simulink model "PowerConverters"  (R2024b)
settings: Solver=FixedStepAuto  StartTime=0.0  StopTime=tfinal  RelTol=1e-4  EnableMultiTasking=on
PreLoadFcn:
  | PowerConvertersInit;
InitFcn:
  | PowerConvertersInit;
values from neighbouring files (symbols this model uses):
  AmplitudeVar_Buck = 50    [PowerConvertersInit.m]
  Cfilter = 200e-6    (= 0.0002)    [PowerConvertersInit.m]
  Clink_3L = Pnom_dc_3L*H_3L*2 /Vnom_dc_3L^2    (= 0.0666666666667)    [PowerConvertersInit.m]
  Clink_stat = Pnom_stat*H_stat*2 /Vnom_dc_stat^2    (= 0.0115740740741)    [PowerConvertersInit.m]
  D_Boost = 0.8    [PowerConvertersInit.m]
  D_Buck = 0.55    [PowerConvertersInit.m]
  Fnom = 60    [PowerConvertersInit.m]
  FrequencyVar_Buck = 5    [PowerConvertersInit.m]
  Fsys_FB = 50    [PowerConvertersInit.m]
  J = 10    [PowerConvertersInit.m]
  Ki_Ireg_3L = 8    [PowerConvertersInit.m]
  Ki_Ireg_motor = 0.25    [PowerConvertersInit.m]
  Ki_Ireg_stat = 80    [PowerConvertersInit.m]
  Ki_VDCreg_3L = 275    [PowerConvertersInit.m]
  Ki_VDCreg_stat = 800    [PowerConvertersInit.m]
  Ki_wreg_motor = 50    [PowerConvertersInit.m]
  Kp_Ireg_3L = 0.2/2    (= 0.1)    [PowerConvertersInit.m]
  Kp_Ireg_motor = 0.0015    [PowerConvertersInit.m]
  Kp_Ireg_stat = 0.35    [PowerConvertersInit.m]
  Kp_VDCreg_3L = 2.5    [PowerConvertersInit.m]
  Kp_VDCreg_stat = 10    [PowerConvertersInit.m]
  Kp_wreg_motor = 15    [PowerConvertersInit.m]
  Lchoke_Boost = 1e-3    (= 0.001)    [PowerConvertersInit.m]
  Lchoke_Buck = 5e-3    (= 0.005)    [PowerConvertersInit.m]
  Lchoke_FB = 1e-3    (= 0.001)    [PowerConvertersInit.m]
  Lff_3L = Lxfo_3L    (= 0.1)    [PowerConvertersInit.m]
  Lff_stat = Lxfo_Tr_stat+0.06*2    (= 0.18)    [PowerConvertersInit.m]
  Limit_Ireg_motor = [1, 0]    [PowerConvertersInit.m]
  Limit_wreg_motor = [1000, -1000]    [PowerConvertersInit.m]
  LimitL_Ireg_3L = -1.5    [PowerConvertersInit.m]
  LimitL_Ireg_stat = -1.5    [PowerConvertersInit.m]
  LimitL_VDCreg_3L = -1.5    [PowerConvertersInit.m]
  LimitL_VDCreg_stat = -1.5    [PowerConvertersInit.m]
  LimitU_Ireg_3L = 1.5    [PowerConvertersInit.m]
  LimitU_Ireg_stat = 1.5    [PowerConvertersInit.m]
  LimitU_VDCreg_3L = 1.5    [PowerConvertersInit.m]
  LimitU_VDCreg_stat = 1.5    [PowerConvertersInit.m]
  Lm_Tr_stat = 200    [PowerConvertersInit.m]
  Lstat = 0.1*Lbase_sec    (= 0.000671434916169)    [PowerConvertersInit.m]
  Lxfo_3L = 0.10    (= 0.1)    [PowerConvertersInit.m]
  Lxfo_Tr_stat = 0.06    [PowerConvertersInit.m]
  m_FB = 0.9    [PowerConvertersInit.m]
  m_HB = 1    [PowerConvertersInit.m]
  Pnom_3L = Pnom_dc_3L    (= 1000000)    [PowerConvertersInit.m]
  Pnom_dc_3L = 1e6    (= 1000000)    [PowerConvertersInit.m]
  Pnom_stat = 2e6    (= 2000000)    [PowerConvertersInit.m]
  Psc_grid = 100e6    (= 100000000)    [PowerConvertersInit.m]
  R_DCsrc = 0.5    [PowerConvertersInit.m]
  RateLimit_Iref_motor = 20000    [PowerConvertersInit.m]
  RateLimit_Qstat = Fnom*2    (= 120)    [PowerConvertersInit.m]
  RateLimit_wref_motor = 2000    [PowerConvertersInit.m]
  Rchoke_Boost = 50e-3    (= 0.05)    [PowerConvertersInit.m]
  Rchoke_Buck = 10e-3    (= 0.01)    [PowerConvertersInit.m]
  Rchoke_FB = 50e-3    (= 0.05)    [PowerConvertersInit.m]
  Rff_3L = Rxfo_3L    (= 0.00333333333333)    [PowerConvertersInit.m]
  Rff_stat = Rxfo_Tr_stat+0.06/100*2    (= 0.0032)    [PowerConvertersInit.m]
  Rfilter = 1/(Cfilter*377)/50    (= 0.26525198939)    [PowerConvertersInit.m]
  Rload_Buck = 0.1    [PowerConvertersInit.m]
  Rm_Tr_stat = 200    [PowerConvertersInit.m]
  Rstat = Lstat*(2*pi*Fnom)/100    (= 0.00253125)    [PowerConvertersInit.m]
  Rxfo_3L = 0.10/30    (= 0.00333333333333)    [PowerConvertersInit.m]
  Rxfo_Tr_stat = 0.06/30    (= 0.002)    [PowerConvertersInit.m]
  Tload = 1000    [PowerConvertersInit.m]
  Ts_Control = 50e-6    (= 5e-05)    [PowerConvertersInit.m]
  Ts_Power = 1e-7    (= 1e-07)    [PowerConvertersInit.m]
  Ts_PWM = 1e-7    (= 1e-07)    [PowerConvertersInit.m]
  V_DCsrc = 500    [PowerConvertersInit.m]
  Vload_Buck = 500    [PowerConvertersInit.m]
  Vnom_dc_3L = 1000    [PowerConvertersInit.m]
  Vnom_dc_stat = 2400    [PowerConvertersInit.m]
  Vnom_grid = 25e3    (= 25000)    [PowerConvertersInit.m]
  Vnom_prim_3L = Vnom_grid    (= 25000)    [PowerConvertersInit.m]
  Vnom_prim_stat = Vnom_grid    (= 25000)    [PowerConvertersInit.m]
  Vnom_sec_3L = 0.5*Vnom_dc_3L/sqrt(2)*sqrt(3)*m_nom_3L    [PowerConvertersInit.m]
  Vnom_sec_stat = 1800*1.25    (= 2250)    [PowerConvertersInit.m]
  wref_Initial = w_Initial*30/pi    (= 1200)    [PowerConvertersInit.m]
undefined symbols (not defined in the file or in its folder): D1, Delta, DiscIntNeverNeededParam
libraries: spsSeriesRLCBranchLib x21, spsVoltageMeasurementLib x9, spsPWMGeneratorPulseAveragingLib x7, spsCurrentMeasurementLib x5, spsMeanLib x5, spsPWMGenerator2LevelLib x4, spsPWMGeneratorDCDCLib x4, spsabctodq0Lib x4, spsSecondOrderFilterLib x4, spsLinearTransformerLib x3, spsThreePhaseVIMeasurementLib x3, spsSeriesRLCLoadLib x2
(part 2 of 2)

== system PowerConverters/Control Systems/PWM Gen Boost ==
  Select : Inport
  D : Inport  Port=2
  PWM Gen : Subsystem
  Switch1 : Switch  Threshold=1.5  SaturateOnIntegerOverflow=off  InputSameDT=off
  g : Outport  VectorParamsAs1DForOutWhenUnconnected=off
  wires:
  D/1 -> PWM Gen/1(D)
  Select/1 -> Switch1/2, PWM Gen/Enable
  Switch1/1 -> g/1
  PWM Gen/1(g) -> Switch1/3
  PWM Gen/2(g_Pavg) -> Switch1/1

== system PowerConverters/Control Systems/PWM Gen Buck ==
  Select : Inport
  D : Inport  Port=2
  PWM Gen : Subsystem
  Switch1 : Switch  Threshold=1.5  SaturateOnIntegerOverflow=off  InputSameDT=off
  g : Outport  VectorParamsAs1DForOutWhenUnconnected=off
  wires:
  PWM Gen/2(g_Pavg) -> Switch1/1
  PWM Gen/1(g) -> Switch1/3
  Switch1/1 -> g/1
  Select/1 -> PWM Gen/Enable, Switch1/2
  D/1 -> PWM Gen/1(D)

== system PowerConverters/Control Systems/PWM Gen FB ==
  Select : Inport
  Uref : Inport  Port=2
  PWM gen : Subsystem
  Switch1 : Switch  Threshold=1.5  SaturateOnIntegerOverflow=off  InputSameDT=off
  g : Outport  VectorParamsAs1DForOutWhenUnconnected=off
  wires:
  PWM gen/1(g) -> Switch1/3
  Switch1/1 -> g/1
  Select/1 -> PWM gen/Enable, Switch1/2
  Uref/1 -> PWM gen/1(Uref)
  PWM gen/2(g_Pavg) -> Switch1/1

== system PowerConverters/Control Systems/PWM Gen HB ==
  Select : Inport
  Uref : Inport  Port=2
  Subsystem : Subsystem
  Switch1 : Switch  Threshold=1.5  SaturateOnIntegerOverflow=off  InputSameDT=off
  g : Outport  VectorParamsAs1DForOutWhenUnconnected=off
  wires:
  Uref/1 -> Subsystem/1(Uref)
  Select/1 -> Switch1/2, Subsystem/Enable
  Switch1/1 -> g/1
  Subsystem/1(g) -> Switch1/3
  Subsystem/2(g_Pavg) -> Switch1/1

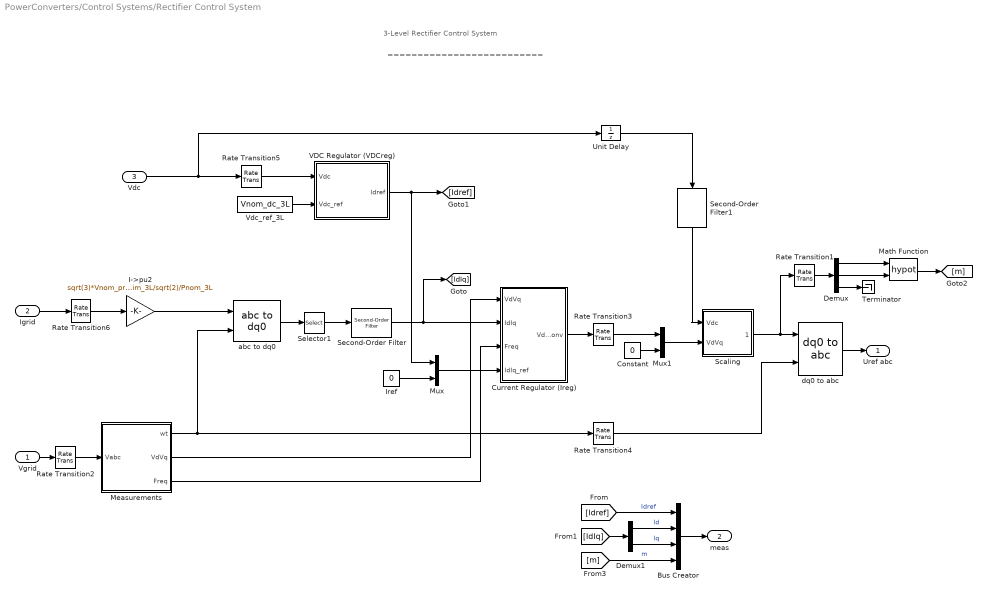
== system PowerConverters/Control Systems/Rectifier Control System ==
  note: 3-Level Rectifier Control System
  note: ==========================
  Vgrid : Inport  PortDimensions=3
  Igrid : Inport  Port=2  PortDimensions=3
  Vdc : Inport  Port=3
  Bus Creator : BusCreator  Inputs=4
  Constant : Constant  Value=0
  Current Regulator (Ireg) : Subsystem
  Demux : Demux  Outputs=3
  Demux1 : Demux  Outputs=2
  I->pu2 : Gain  Gain=sqrt(3)*Vnom_prim_3L/sqrt(2)/Pnom_3L  SaturateOnIntegerOverflow=on  OutDataTypeStr=Inherit: Same as input  ParamDataTypeStr=Inherit: Same as input
  Iref : Constant  Value=0
  Math Function : Math  Operator=hypot  SignedPower=on
  Measurements : Subsystem
  Mux : Mux  Inputs=2
  Mux1 : Mux  Inputs=[2 1]
  Rate Transition{1..2,5..6} (4 alike) : RateTransition  OutPortSampleTime=Ts_Control
  Rate Transition3 : RateTransition  OutPortSampleTime=Ts_PWM
  Rate Transition4 : RateTransition  OutPortSampleTime=Ts_PWM
  Scaling : Subsystem
  Second-Order Filter : spsSecondOrderFilterLib/Second-Order Filter  FilterType=Lowpass  Fo=Freq_Filter  Zeta=1  Ts=Ts_Control  Initialize=off  Vac_Init="[0,  0,  60]"  Vdc_Init=0  PlotResponse=off  FreqRange=[0, 500, 1]
  Second-Order Filter1 : spsSecondOrderFilterLib/Second-Order Filter  FilterType=Lowpass  Fo=Freq_Filter  Zeta=1  Ts=Ts_PWM  Initialize=off  Vac_Init="[0,  0,  60]"  Vdc_Init=0  PlotResponse=off  FreqRange=[0, 500, 1]
  Selector1 : Selector  InputPortWidth=3  IndexOptions=Index vector (dialog)  Indices=[1 2]  OutputSizes=1
  Terminator : Terminator
  Unit Delay : UnitDelay  SampleTime=Ts_PWM  HasFrameUpgradeWarning=on
  VDC Regulator (VDCreg) : Subsystem
  Vdc_ref_3L : Constant  Value=Vnom_dc_3L
  abc to dq0 : spsabctodq0Lib/abc to dq0  Alignment=90 degrees behind phase A axis
  dq0 to abc : spsdq0toabcLib/dq0 to abc  Alignment=90 degrees behind phase A axis
  Uref abc : Outport  VectorParamsAs1DForOutWhenUnconnected=off
  meas : Outport  Port=2  VectorParamsAs1DForOutWhenUnconnected=off
  wires:
  Selector1/1 -> Second-Order Filter/1
  I->pu2/1 -> abc to dq0/1
  Igrid/1 -> Rate Transition6/1
  abc to dq0/1 -> Selector1/1
  VDC Regulator (VDCreg)/1(Idref) -> [Idref], Mux/1
  Scaling/1(VdVq*) -> dq0 to abc/1, Rate Transition1/1
  Mux1/1 -> Scaling/2(VdVq)
  Mux/1 -> Current Regulator (Ireg)/4(IdIq_ref)
  Demux/3 -> Terminator/1
  Demux/2 -> Math Function/2
  Demux/1 -> Math Function/1
  Constant/1 -> Mux1/2
  Rate Transition3/1 -> Mux1/1
  Rate Transition4/1 -> dq0 to abc/2
  Current Regulator (Ireg)/1(VdVq_conv) -> Rate Transition3/1
  dq0 to abc/1 -> Uref abc/1
  Vgrid/1 -> Rate Transition2/1
  Rate Transition2/1 -> Measurements/1(Vabc)
  Rate Transition6/1 -> I->pu2/1
  Measurements/1(wt) -> Rate Transition4/1, abc to dq0/2
  Measurements/2(VdVq) -> Current Regulator (Ireg)/1(VdVq)
  Measurements/3(Freq) -> Current Regulator (Ireg)/3(Freq)
  Iref/1 -> Mux/2
  Vdc_ref_3L/1 -> VDC Regulator (VDCreg)/2(Vdc_ref)
  [Idref] -> Bus Creator/1  "Idref"
  Demux1/1 -> Bus Creator/2  "Id"
  Demux1/2 -> Bus Creator/3  "Iq"
  [m] -> Bus Creator/4  "m"
  [IdIq] -> Demux1/1
  Bus Creator/1 -> meas/1
  Math Function/1 -> [m]
  Rate Transition5/1 -> VDC Regulator (VDCreg)/1(Vdc)
  Rate Transition1/1 -> Demux/1
  Vdc/1 -> Unit Delay/1, Rate Transition5/1
  Unit Delay/1 -> Second-Order Filter1/1
  Second-Order Filter/1 -> [IdIq], Current Regulator (Ireg)/2(IdIq)
  Second-Order Filter1/1 -> Scaling/1(Vdc)

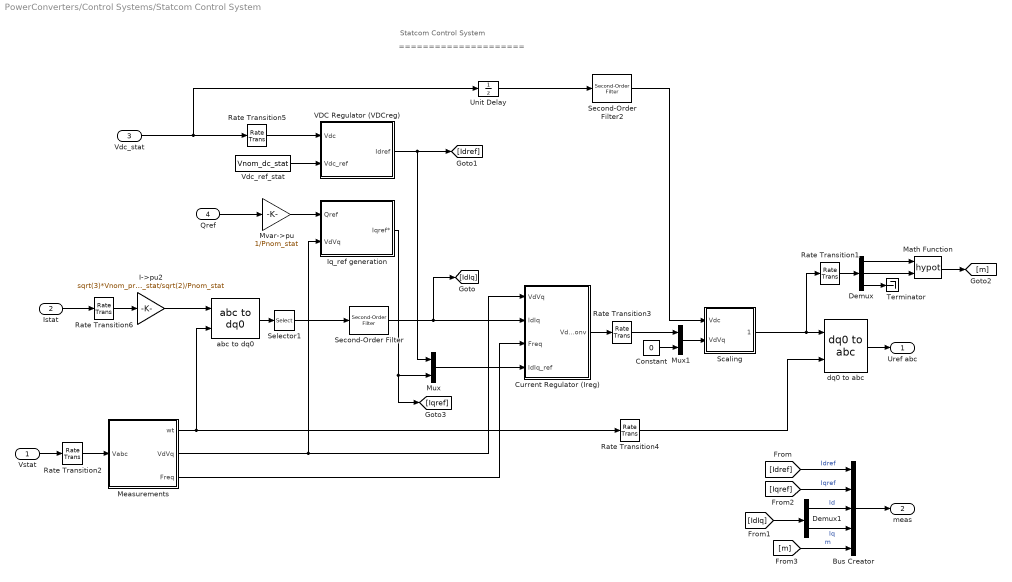
== system PowerConverters/Control Systems/Statcom Control System ==
  note: Statcom Control System
  note: =====================
  Vstat : Inport  PortDimensions=3
  Istat : Inport  Port=2  PortDimensions=3
  Vdc_stat : Inport  Port=3
  Qref : Inport  Port=4  PortDimensions=1
  Bus Creator : BusCreator  Inputs=5
  Constant : Constant  Value=0
  Current Regulator (Ireg) : Subsystem
  Demux : Demux  Outputs=3
  Demux1 : Demux  Outputs=2
  I->pu2 : Gain  Gain=sqrt(3)*Vnom_prim_stat/sqrt(2)/Pnom_stat  SaturateOnIntegerOverflow=on  OutDataTypeStr=Inherit: Same as input  ParamDataTypeStr=Inherit: Same as input
  Iq_ref generation : Subsystem
  Math Function : Math  Operator=hypot  SignedPower=on
  Measurements : Subsystem
  Mux : Mux  Inputs=2
  Mux1 : Mux  Inputs=[2 1]
  Mvar->pu : Gain  Gain=1/Pnom_stat  SaturateOnIntegerOverflow=on  OutDataTypeStr=Inherit: Same as input  ParamDataTypeStr=Inherit: Same as input
  Rate Transition{1..2,5..6} (4 alike) : RateTransition  OutPortSampleTime=Ts_Control
  Rate Transition3 : RateTransition  OutPortSampleTime=Ts_PWM
  Rate Transition4 : RateTransition  OutPortSampleTime=Ts_PWM
  Scaling : Subsystem
  Second-Order Filter : spsSecondOrderFilterLib/Second-Order Filter  FilterType=Lowpass  Fo=Freq_Filter_stat  Zeta=1  Ts=Ts_Control  Initialize=off  Vac_Init="[0,  0,  60]"  Vdc_Init=0  PlotResponse=off  FreqRange=[0, 500, 1]
  Second-Order Filter2 : spsSecondOrderFilterLib/Second-Order Filter  FilterType=Lowpass  Fo=Freq_Filter_stat  Zeta=1  Ts=Ts_PWM  Initialize=off  Vac_Init="[0,  0,  60]"  Vdc_Init=0  PlotResponse=off  FreqRange=[0, 500, 1]
  Selector1 : Selector  InputPortWidth=3  IndexOptions=Index vector (dialog)  Indices=[1 2]  OutputSizes=1
  Terminator : Terminator
  Unit Delay : UnitDelay  SampleTime=Ts_PWM  HasFrameUpgradeWarning=on
  VDC Regulator (VDCreg) : Subsystem
  Vdc_ref_stat : Constant  Value=Vnom_dc_stat
  abc to dq0 : spsabctodq0Lib/abc to dq0  Alignment=90 degrees behind phase A axis
  dq0 to abc : spsdq0toabcLib/dq0 to abc  Alignment=90 degrees behind phase A axis
  Uref abc : Outport  VectorParamsAs1DForOutWhenUnconnected=off
  meas : Outport  Port=2  VectorParamsAs1DForOutWhenUnconnected=off
  wires:
  Mvar->pu/1 -> Iq_ref generation/1(Qref)
  Second-Order Filter2/1 -> Scaling/1(Vdc)
  Qref/1 -> Mvar->pu/1
  Iq_ref generation/1(Iqref*) -> [Iqref], Mux/2
  Vdc_ref_stat/1 -> VDC Regulator (VDCreg)/2(Vdc_ref)
  VDC Regulator (VDCreg)/1(Idref) -> [Idref], Mux/1
  [m] -> Bus Creator/5  "m"
  Demux1/2 -> Bus Creator/4  "Iq"
  Demux1/1 -> Bus Creator/3  "Id"
  [Iqref] -> Bus Creator/2  "Iqref"
  [Idref] -> Bus Creator/1  "Idref"
  Selector1/1 -> Second-Order Filter/1
  I->pu2/1 -> abc to dq0/1
  Istat/1 -> Rate Transition6/1
  abc to dq0/1 -> Selector1/1
  Scaling/1(VdVq*) -> dq0 to abc/1, Rate Transition1/1
  Mux1/1 -> Scaling/2(VdVq)
  Mux/1 -> Current Regulator (Ireg)/4(IdIq_ref)
  Demux/3 -> Terminator/1
  Demux/2 -> Math Function/2
  Demux/1 -> Math Function/1
  Constant/1 -> Mux1/2
  Rate Transition3/1 -> Mux1/1
  Rate Transition4/1 -> dq0 to abc/2
  Current Regulator (Ireg)/1(VdVq_conv) -> Rate Transition3/1
  dq0 to abc/1 -> Uref abc/1
  Vstat/1 -> Rate Transition2/1
  Rate Transition2/1 -> Measurements/1(Vabc)
  Rate Transition6/1 -> I->pu2/1
  Measurements/1(wt) -> Rate Transition4/1, abc to dq0/2
  Measurements/2(VdVq) -> Iq_ref generation/2(VdVq), Current Regulator (Ireg)/1(VdVq)
  Measurements/3(Freq) -> Current Regulator (Ireg)/3(Freq)
  [IdIq] -> Demux1/1
  Bus Creator/1 -> meas/1
  Math Function/1 -> [m]
  Rate Transition5/1 -> VDC Regulator (VDCreg)/1(Vdc)
  Rate Transition1/1 -> Demux/1
  Vdc_stat/1 -> Unit Delay/1, Rate Transition5/1
  Second-Order Filter/1 -> [IdIq], Current Regulator (Ireg)/2(IdIq)
  Unit Delay/1 -> Second-Order Filter2/1

== system PowerConverters/Control Systems/DC Motor Control/Current regulator Ireg_motor ==
  Error : Inport  SampleTime=Ts
  Discrete-Time Integrator : DiscreteIntegrator  InitialCondition=Init  SampleTime=Ts  LimitOutput=on  UpperSaturationLimit=UpperLimit  LowerSaturationLimit=LowerLimit  ICPrevOutput=DiscIntNeverNeededParam  ICPrevScaledInput=DiscIntNeverNeededParam
  Kp4 : Gain  Gain=Kp  SaturateOnIntegerOverflow=on  SampleTime=Ts  OutDataTypeStr=Inherit: Same as input  ParamDataTypeStr=Inherit: Same as input
  Kp5 : Gain  Gain=Ki  SaturateOnIntegerOverflow=on  SampleTime=Ts  OutDataTypeStr=Inherit: Same as input  ParamDataTypeStr=Inherit: Same as input
  Saturation2 : Saturate  UpperLimit=UpperLimit  LowerLimit=LowerLimit  SampleTime=Ts
  Sum6 : Sum  InputSameDT=on  SaturateOnIntegerOverflow=on  SampleTime=Ts  OutDataTypeStr=Inherit: Same as first input
  Zero-Order Hold : ZeroOrderHold  SampleTime=Ts
  Out : Outport  SampleTime=Ts  InitialOutput=0  VectorParamsAs1DForOutWhenUnconnected=off
  wires:
  Zero-Order Hold/1 -> Sum6/1
  Saturation2/1 -> Out/1
  Discrete-Time Integrator/1 -> Sum6/2
  Kp4/1 -> Zero-Order Hold/1
  Kp5/1 -> Discrete-Time Integrator/1
  Sum6/1 -> Saturation2/1
  Error/1 -> Kp5/1, Kp4/1

== system PowerConverters/Control Systems/DC Motor Control/Speed Regulator wreg ==
  Error : Inport  SampleTime=Ts
  Discrete-Time Integrator : DiscreteIntegrator  InitialCondition=Init  SampleTime=Ts  LimitOutput=on  UpperSaturationLimit=UpperLimit  LowerSaturationLimit=LowerLimit  ICPrevOutput=DiscIntNeverNeededParam  ICPrevScaledInput=DiscIntNeverNeededParam
  Kp4 : Gain  Gain=Kp  SaturateOnIntegerOverflow=on  SampleTime=Ts  OutDataTypeStr=Inherit: Same as input  ParamDataTypeStr=Inherit: Same as input
  Kp5 : Gain  Gain=Ki  SaturateOnIntegerOverflow=on  SampleTime=Ts  OutDataTypeStr=Inherit: Same as input  ParamDataTypeStr=Inherit: Same as input
  Saturation2 : Saturate  UpperLimit=UpperLimit  LowerLimit=LowerLimit  SampleTime=Ts
  Sum6 : Sum  InputSameDT=on  SaturateOnIntegerOverflow=on  SampleTime=Ts  OutDataTypeStr=Inherit: Same as first input
  Zero-Order Hold : ZeroOrderHold  SampleTime=Ts
  Out : Outport  SampleTime=Ts  InitialOutput=0  VectorParamsAs1DForOutWhenUnconnected=off
  wires:
  Zero-Order Hold/1 -> Sum6/1
  Saturation2/1 -> Out/1
  Discrete-Time Integrator/1 -> Sum6/2
  Kp4/1 -> Zero-Order Hold/1
  Kp5/1 -> Discrete-Time Integrator/1
  Sum6/1 -> Saturation2/1
  Error/1 -> Kp5/1, Kp4/1

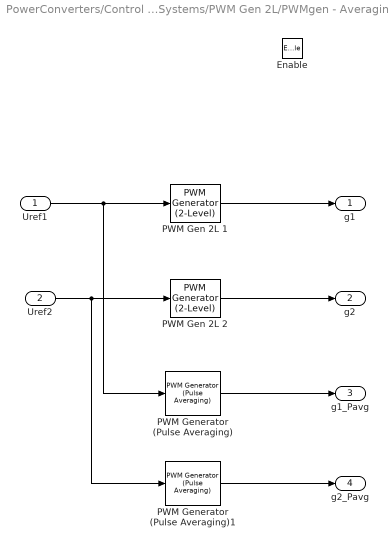
== system PowerConverters/Control Systems/PWM Gen 2L/PWMgen - Averaging ==
  Uref1 : Inport
  Uref2 : Inport  Port=2
  Enable : EnablePort
  PWM Gen 2L 1 : spsPWMGenerator2LevelLib/PWM Generator (2-Level)  ModulatorType=Three-phase bridge (6 pulses)  ModulatorMode=Unsynchronized  Fc=Fc_stat  Pc=90  nF=27  MinMax="[ -1  1 ]"  SamplingTechnique=Natural  ModulatingSignals=off  m=0.8  Freq=60  Phase=0  Ts=Ts_PWM  ShowCarrierOutport=off
  PWM Gen 2L 2 : spsPWMGenerator2LevelLib/PWM Generator (2-Level)  ModulatorType=Three-phase bridge (6 pulses)  ModulatorMode=Unsynchronized  Fc=Fc_stat  Pc=90  nF=27  MinMax="[ -1  1 ]"  SamplingTechnique=Natural  ModulatingSignals=off  m=0.8  Freq=60  Phase=0  Ts=Ts_PWM  ShowCarrierOutport=off
  PWM Generator (Pulse Averaging) : spsPWMGeneratorPulseAveragingLib/PWM Generator (Pulse Averaging)  GeneratorType=Two-level, three-phase  Fc=Fc_stat  InitialPhase=90  Ts=Ts_PWM
  PWM Generator (Pulse Averaging)1 : spsPWMGeneratorPulseAveragingLib/PWM Generator (Pulse Averaging)  GeneratorType=Two-level, three-phase  Fc=Fc_stat  InitialPhase=90  Ts=Ts_PWM
  g1 : Outport  VectorParamsAs1DForOutWhenUnconnected=off
  g2 : Outport  Port=2  VectorParamsAs1DForOutWhenUnconnected=off
  g1_Pavg : Outport  Port=3  VectorParamsAs1DForOutWhenUnconnected=off
  g2_Pavg : Outport  Port=4  VectorParamsAs1DForOutWhenUnconnected=off
  wires:
  Uref1/1 -> PWM Generator (Pulse Averaging)/1, PWM Gen 2L 1/1
  Uref2/1 -> PWM Generator (Pulse Averaging)1/1, PWM Gen 2L 2/1
  PWM Gen 2L 1/1 -> g1/1
  PWM Gen 2L 2/1 -> g2/1
  PWM Generator (Pulse Averaging)/1 -> g1_Pavg/1
  PWM Generator (Pulse Averaging)1/1 -> g2_Pavg/1

== system PowerConverters/Control Systems/PWM Gen 2Q/Subsystem ==
  D : Inport
  Enable : EnablePort
  Logical Operator : Logic  Operator=NOT  AllPortsSameDT=off  OutDataTypeStr=float('double')
  Mux : Mux  Inputs=2
  "PWM Gen 2Q " : spsPWMGeneratorDCDCLib/PWM Generator (DC-DC)  Fsw=Fc_motor  Ts=Ts_PWM
  PWM Generator (Pulse Averaging) : spsPWMGeneratorPulseAveragingLib/PWM Generator (Pulse Averaging)  GeneratorType=Two-quadrant  Fc=Fc_motor  InitialPhase=0  Ts=Ts_PWM
  g : Outport  VectorParamsAs1DForOutWhenUnconnected=off
  g_Pavg : Outport  Port=2  VectorParamsAs1DForOutWhenUnconnected=off
  wires:
  Mux/1 -> g/1
  Logical Operator/1 -> Mux/2
  D/1 -> PWM Generator (Pulse Averaging)/1, "PWM Gen 2Q "/1
  "PWM Gen 2Q "/1 -> Logical Operator/1, Mux/1
  PWM Generator (Pulse Averaging)/1 -> g_Pavg/1

== system PowerConverters/Control Systems/PWM Gen 3L/PWMgen - Averaging ==
  Uref : Inport
  Enable : EnablePort
  PWM Generator (Pulse Averaging) : spsPWMGeneratorPulseAveragingLib/PWM Generator (Pulse Averaging)  GeneratorType=Three-level, three-phase  Fc=Fc_3L  InitialPhase=0  Ts=Ts_PWM
  Subsystem : Subsystem
  Pavg : Outport  VectorParamsAs1DForOutWhenUnconnected=off
  P : Outport  Port=2  VectorParamsAs1DForOutWhenUnconnected=off
  wires:
  Uref/1 -> Subsystem/1(Uref), PWM Generator (Pulse Averaging)/1
  PWM Generator (Pulse Averaging)/1 -> Pavg/1
  Subsystem/1(P) -> P/1

== system PowerConverters/Control Systems/PWM Gen Boost/PWM Gen ==
  D : Inport
  Enable : EnablePort
  "PWM Gen Buck " : spsPWMGeneratorDCDCLib/PWM Generator (DC-DC)  Fsw=Fc_Boost  Ts=Ts_PWM
  PWM Generator (DC-DC) : spsPWMGeneratorDCDCLib/PWM Generator (DC-DC)  Fsw=Fc_Boost  Ts=Ts_PWM
  g : Outport  VectorParamsAs1DForOutWhenUnconnected=off
  g_Pavg : Outport  Port=2  VectorParamsAs1DForOutWhenUnconnected=off
  wires:
  "PWM Gen Buck "/1 -> g/1
  D/1 -> PWM Generator (DC-DC)/1, "PWM Gen Buck "/1
  PWM Generator (DC-DC)/1 -> g_Pavg/1

== system PowerConverters/Control Systems/PWM Gen Buck/PWM Gen ==
  D : Inport
  Enable : EnablePort
  "PWM Gen Buck " : spsPWMGeneratorDCDCLib/PWM Generator (DC-DC)  Fsw=Fc_Buck  Ts=Ts_PWM
  PWM Generator (Pulse Averaging) : spsPWMGeneratorPulseAveragingLib/PWM Generator (Pulse Averaging)  GeneratorType=Two-quadrant  Fc=Fc_Buck  InitialPhase=0  Ts=Ts_PWM
  Selector : Selector  InputPortWidth=2  IndexOptions=Index vector (dialog)  Indices=1  OutputSizes=1
  g : Outport  VectorParamsAs1DForOutWhenUnconnected=off
  g_Pavg : Outport  Port=2  VectorParamsAs1DForOutWhenUnconnected=off
  wires:
  PWM Generator (Pulse Averaging)/1 -> Selector/1
  D/1 -> PWM Generator (Pulse Averaging)/1, "PWM Gen Buck "/1
  "PWM Gen Buck "/1 -> g/1
  Selector/1 -> g_Pavg/1

== system PowerConverters/Control Systems/PWM Gen FB/PWM gen ==
  Uref : Inport
  Enable : EnablePort
  PWM Gen FB : spsPWMGenerator2LevelLib/PWM Generator (2-Level)  ModulatorType=Single-phase full-bridge (4 pulses)  ModulatorMode=Unsynchronized  Fc=Fc_FB  Pc=90  nF=27  MinMax="[ -1  1 ]"  SamplingTechnique=Natural  ModulatingSignals=off  m=0.8  Freq=60  Phase=0  Ts=Ts_PWM  ShowCarrierOutport=off
  PWM Generator (Pulse Averaging) : spsPWMGeneratorPulseAveragingLib/PWM Generator (Pulse Averaging)  GeneratorType=Full-bridge, single phase  Fc=Fc_FB  InitialPhase=90  Ts=Ts_PWM
  g : Outport  VectorParamsAs1DForOutWhenUnconnected=off
  g_Pavg : Outport  Port=2  VectorParamsAs1DForOutWhenUnconnected=off
  wires:
  PWM Generator (Pulse Averaging)/1 -> g_Pavg/1
  PWM Gen FB/1 -> g/1
  Uref/1 -> PWM Generator (Pulse Averaging)/1, PWM Gen FB/1

== system PowerConverters/Control Systems/PWM Gen HB/Subsystem ==
  Uref : Inport
  Enable : EnablePort
  PWM Gen HB : spsPWMGenerator2LevelLib/PWM Generator (2-Level)  ModulatorType=Single-phase half-bridge (2 pulses)  ModulatorMode=Unsynchronized  Fc=Fc_HB  Pc=90  nF=27  MinMax="[ -1  1 ]"  SamplingTechnique=Natural  ModulatingSignals=off  m=0.8  Freq=60  Phase=0  Ts=Ts_PWM  ShowCarrierOutport=off
  PWM Generator (Pulse Averaging) : spsPWMGeneratorPulseAveragingLib/PWM Generator (Pulse Averaging)  GeneratorType=Full-bridge, single phase  Fc=Fc_HB  InitialPhase=0  Ts=Ts_PWM
  Selector : Selector  InputPortWidth=4  IndexOptions=Index vector (dialog)  Indices=[1,2]  OutputSizes=1
  g : Outport  VectorParamsAs1DForOutWhenUnconnected=off
  g_Pavg : Outport  Port=2  VectorParamsAs1DForOutWhenUnconnected=off
  wires:
  PWM Gen HB/1 -> g/1
  Selector/1 -> g_Pavg/1
  PWM Generator (Pulse Averaging)/1 -> Selector/1
  Uref/1 -> PWM Generator (Pulse Averaging)/1, PWM Gen HB/1

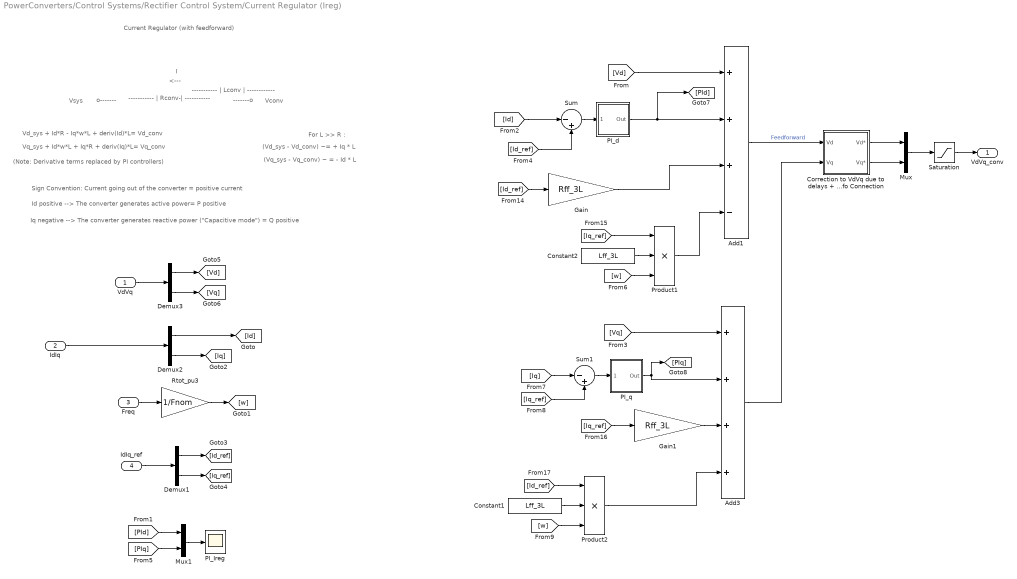
== system PowerConverters/Control Systems/Rectifier Control System/Current Regulator (Ireg) ==
  note: <---
  note: -------o
  note: Vconv
  note: -----------
      | | Lconv |
      | ------------
  note: ----
  note: -----------
      | | Rconv |
      | -----------
  note: For L >> R :
  note: (Vq_sys - Vq_conv) ~ = - Id * L
  note: (Vd_sys - Vd_conv) ~= + Iq * L
  note: Id positive --> The converter generates active power= P positive
  note: Iq negative --> The converter generates reactive power ("Capacitive mode") = Q positive
  note: Sign Convention: Current going out of the converter = positive current
  note: Current Regulator
      | (with feedforward)
  note: Vq_sys + Id*w*L + Iq*R + deriv(Iq)*L= Vq_conv
  note: Vd_sys + Id*R - Iq*w*L + deriv(Id)*L= Vd_conv
  note: (Note: Derivative terms replaced by PI controllers)
  note: Vsys
  note: o-------
  note: I
  VdVq : Inport  PortDimensions=2
  IdIq : Inport  Port=2  PortDimensions=2
  Freq : Inport  Port=3  PortDimensions=1
  IdIq_ref : Inport  Port=4  PortDimensions=2
  Add1 : Sum  Inputs=+++-
  Add3 : Sum  Inputs=++++
  Constant1 : Constant  Value=Lff_3L  SampleTime=Ts_Control
  Constant2 : Constant  Value=Lff_3L  SampleTime=Ts_Control
  Correction to VdVq due to delays + Transfo Connection : Subsystem
  Demux1 : Demux  Outputs=2
  Demux2 : Demux  Outputs=2
  Demux3 : Demux  Outputs=2
  Gain : Gain  Gain=Rff_3L
  Gain1 : Gain  Gain=Rff_3L
  Mux : Mux  Inputs=2
  Mux1 : Mux  Inputs=2
  PI_Ireg : Scope
  PI_d : Subsystem  DialogController=POWERSYS.PowerSysDialog  mask(Discrete PI Controller){Kp=Kp_Ireg_3L, Ki=Ki_Ireg_3L, Par_Limits=[ LimitU_Ireg_3L LimitL_Ireg_3L ], Init=0, Ts=Ts_Control}
      mask prompts: Kp "Proportional gain (Kp):"; Ki "Integral gain (Ki):"; Par_Limits "Output limits: [ Upper   Lower ]"; Init "Output initial value:"; Ts "Sample time:"
      mask help: This block implements a discrete PI controller.
      mask init:
      | UpperLimit=Par_Limits(1);
      | LowerLimit=Par_Limits(2);
      mask Display: disp('PI');
  PI_q : Subsystem  DialogController=POWERSYS.PowerSysDialog  mask(Discrete PI Controller){Kp=Kp_Ireg_3L, Ki=Ki_Ireg_3L, Par_Limits=[ LimitU_Ireg_3L LimitL_Ireg_3L ], Init=0, Ts=Ts_Control}
      mask prompts: Kp "Proportional gain (Kp):"; Ki "Integral gain (Ki):"; Par_Limits "Output limits: [ Upper   Lower ]"; Init "Output initial value:"; Ts "Sample time:"
      mask help: This block implements a discrete PI controller.
      mask init:
      | UpperLimit=Par_Limits(1);
      | LowerLimit=Par_Limits(2);
      mask Display: disp('PI');
  Product1 : Product  Inputs=3  RndMeth=Zero
  Product2 : Product  Inputs=3  RndMeth=Zero
  Rtot_pu3 : Gain  Gain=1/Fnom  SaturateOnIntegerOverflow=on  OutDataTypeStr=Inherit: Same as input  ParamDataTypeStr=Inherit: Same as input
  Saturation : Saturate  UpperLimit=LimitU_Ireg_3L  LowerLimit=LimitL_Ireg_3L
  Sum : Sum  Inputs=|-+
  Sum1 : Sum  Inputs=|-+
  VdVq_conv : Outport  VectorParamsAs1DForOutWhenUnconnected=off
  wires:
  Add3/1 -> Correction to VdVq due to delays + Transfo Connection/2(Vq)
  Add1/1 -> Correction to VdVq due to delays + Transfo Connection/1(Vd)  "Feedforward"
  PI_d/1(Out) -> [PId], Add1/2
  PI_q/1(Out) -> [PIq], Add3/2
  [Vd] -> Add1/1
  Product1/1 -> Add1/4
  Gain/1 -> Add1/3
  Gain1/1 -> Add3/3
  Product2/1 -> Add3/4
  [Vq] -> Add3/1
  Demux2/1 -> [Id]
  IdIq/1 -> Demux2/1
  [Id_ref] -> Product2/1
  [Iq_ref] -> Gain1/1
  [Iq_ref] -> Product1/1
  [Id_ref] -> Gain/1
  Saturation/1 -> VdVq_conv/1
  [Id] -> Sum/1
  [Iq] -> Sum1/1
  Demux2/2 -> [Iq]
  Correction to VdVq due to delays + Transfo Connection/2(Vq*) -> Mux/2
  Correction to VdVq due to delays + Transfo Connection/1(Vd*) -> Mux/1
  [PIq] -> Mux1/2
  [PId] -> Mux1/1
  [w] -> Product1/3
  Constant2/1 -> Product1/2
  [w] -> Product2/3
  Constant1/1 -> Product2/2
  Mux1/1 -> PI_Ireg/1
  [Iq_ref] -> Sum1/2
  Sum1/1 -> PI_q/1(Error)
  [Id_ref] -> Sum/2
  Sum/1 -> PI_d/1(Error)
  Mux/1 -> Saturation/1
  VdVq/1 -> Demux3/1
  Demux3/2 -> [Vq]
  Demux3/1 -> [Vd]
  IdIq_ref/1 -> Demux1/1
  Demux1/2 -> [Iq_ref]
  Demux1/1 -> [Id_ref]
  Rtot_pu3/1 -> [w]
  Freq/1 -> Rtot_pu3/1

== system PowerConverters/Control Systems/Rectifier Control System/Measurements ==
  Vabc : Inport  PortDimensions=3
  PLL (3ph) : spsPLL3phLib/PLL (3ph)  Fmin=45  Par_Init=[0, Fnom]  ParK=[180, 3200, 0]/2  TcD=1e-4  MaxRateChangeFreq=12  FilterCutOffFreq=25  Ts=Ts_Control  AGC=on
  Selector2 : Selector  InputPortWidth=3  IndexOptions=Index vector (dialog)  Indices=[1 2]  OutputSizes=1
  V->pu1 : Gain  Gain=1/(Vnom_prim_3L*sqrt(2)/sqrt(3))  SaturateOnIntegerOverflow=on  OutDataTypeStr=Inherit: Same as input  ParamDataTypeStr=Inherit: Same as input
  abc to dq1 : spsabctodq0Lib/abc to dq0  Alignment=90 degrees behind phase A axis
  wt : Outport  VectorParamsAs1DForOutWhenUnconnected=off
  VdVq : Outport  Port=2  VectorParamsAs1DForOutWhenUnconnected=off
  Freq : Outport  Port=3  VectorParamsAs1DForOutWhenUnconnected=off
  wires:
  Selector2/1 -> VdVq/1
  abc to dq1/1 -> Selector2/1
  PLL (3ph)/1 -> Freq/1
  V->pu1/1 -> PLL (3ph)/1, abc to dq1/1
  Vabc/1 -> V->pu1/1
  PLL (3ph)/2 -> wt/1, abc to dq1/2

== system PowerConverters/Control Systems/Rectifier Control System/Scaling ==
  Vdc : Inport
  VdVq : Inport  Port=2
  0.8 to 1.2 x Vnom_dc : Saturate  UpperLimit=1.5*Vnom_dc_3L  LowerLimit=0.5*Vnom_dc_3L
  Constant1 : Constant  Value=Vnom_sec_3L
  Gain1 : Gain  Gain=0.5/sqrt(2)*sqrt(3)
  Product : Product  Inputs=*/
  Product1 : Product  Inputs=**
  VdVq* : Outport  VectorParamsAs1DForOutWhenUnconnected=off
  wires:
  Product1/1 -> VdVq*/1
  VdVq/1 -> Product1/1
  Vdc/1 -> 0.8 to 1.2 x Vnom_dc/1
  Product/1 -> Product1/2
  0.8 to 1.2 x Vnom_dc/1 -> Gain1/1
  Gain1/1 -> Product/2
  Constant1/1 -> Product/1

== system PowerConverters/Control Systems/Rectifier Control System/VDC Regulator (VDCreg) ==
  Vdc : Inport  PortDimensions=1
  Vdc_ref : Inport  Port=2  PortDimensions=1
  Gain : Gain  Gain=1/(Vnom_dc_3L)
  PI_d : Subsystem  DialogController=POWERSYS.PowerSysDialog  mask(Discrete PI Controller){Kp=Kp_VDCreg_3L, Ki=Ki_VDCreg_3L, Par_Limits=[ LimitU_VDCreg_3L LimitL_VDCreg_3L ], Init=0, Ts=Ts_Control}
      mask prompts: Kp "Proportional gain (Kp):"; Ki "Integral gain (Ki):"; Par_Limits "Output limits: [ Upper   Lower ]"; Init "Output initial value:"; Ts "Sample time:"
      mask help: This block implements a discrete PI controller.
      mask init:
      | UpperLimit=Par_Limits(1);
      | LowerLimit=Par_Limits(2);
      mask Display: disp('PI');
  Sum : Sum  Inputs=|-+
  Idref : Outport  VectorParamsAs1DForOutWhenUnconnected=off
  wires:
  PI_d/1(Out) -> Idref/1
  Gain/1 -> PI_d/1(Error)
  Vdc/1 -> Sum/2
  Vdc_ref/1 -> Sum/1
  Sum/1 -> Gain/1

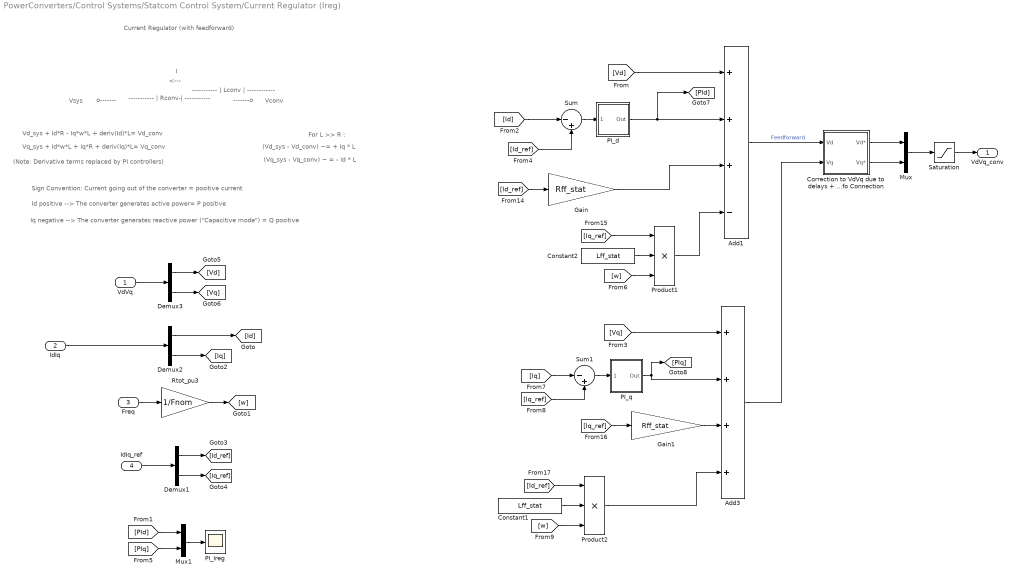
== system PowerConverters/Control Systems/Statcom Control System/Current Regulator (Ireg) ==
  note: <---
  note: -------o
  note: Vconv
  note: -----------
      | | Lconv |
      | ------------
  note: ----
  note: -----------
      | | Rconv |
      | -----------
  note: For L >> R :
  note: (Vq_sys - Vq_conv) ~ = - Id * L
  note: (Vd_sys - Vd_conv) ~= + Iq * L
  note: Id positive --> The converter generates active power= P positive
  note: Iq negative --> The converter generates reactive power ("Capacitive mode") = Q positive
  note: Sign Convention: Current going out of the converter = positive current
  note: Current Regulator
      | (with feedforward)
  note: Vq_sys + Id*w*L + Iq*R + deriv(Iq)*L= Vq_conv
  note: Vd_sys + Id*R - Iq*w*L + deriv(Id)*L= Vd_conv
  note: (Note: Derivative terms replaced by PI controllers)
  note: Vsys
  note: o-------
  note: I
  VdVq : Inport  PortDimensions=2
  IdIq : Inport  Port=2  PortDimensions=2
  Freq : Inport  Port=3  PortDimensions=1
  IdIq_ref : Inport  Port=4  PortDimensions=2
  Add1 : Sum  Inputs=+++-
  Add3 : Sum  Inputs=++++
  Constant1 : Constant  Value=Lff_stat  SampleTime=Ts_Control
  Constant2 : Constant  Value=Lff_stat  SampleTime=Ts_Control
  Correction to VdVq due to delays + Transfo Connection : Subsystem
  Demux1 : Demux  Outputs=2
  Demux2 : Demux  Outputs=2
  Demux3 : Demux  Outputs=2
  Gain : Gain  Gain=Rff_stat
  Gain1 : Gain  Gain=Rff_stat
  Mux : Mux  Inputs=2
  Mux1 : Mux  Inputs=2
  PI_Ireg : Scope
  PI_d : Subsystem  DialogController=POWERSYS.PowerSysDialog  mask(Discrete PI Controller){Kp=Kp_Ireg_stat, Ki=Ki_Ireg_stat, Par_Limits=[ LimitU_Ireg_stat LimitL_Ireg_stat ], Init=0, Ts=Ts_Control}
      mask prompts: Kp "Proportional gain (Kp):"; Ki "Integral gain (Ki):"; Par_Limits "Output limits: [ Upper   Lower ]"; Init "Output initial value:"; Ts "Sample time:"
      mask help: This block implements a discrete PI controller.
      mask init:
      | UpperLimit=Par_Limits(1);
      | LowerLimit=Par_Limits(2);
      mask Display: disp('PI');
  PI_q : Subsystem  DialogController=POWERSYS.PowerSysDialog  mask(Discrete PI Controller){Kp=Kp_Ireg_stat, Ki=Ki_Ireg_stat, Par_Limits=[ LimitU_Ireg_stat LimitL_Ireg_stat ], Init=0, Ts=Ts_Control}
      mask prompts: Kp "Proportional gain (Kp):"; Ki "Integral gain (Ki):"; Par_Limits "Output limits: [ Upper   Lower ]"; Init "Output initial value:"; Ts "Sample time:"
      mask help: This block implements a discrete PI controller.
      mask init:
      | UpperLimit=Par_Limits(1);
      | LowerLimit=Par_Limits(2);
      mask Display: disp('PI');
  Product1 : Product  Inputs=3  RndMeth=Zero
  Product2 : Product  Inputs=3  RndMeth=Zero
  Rtot_pu3 : Gain  Gain=1/Fnom  SaturateOnIntegerOverflow=on  OutDataTypeStr=Inherit: Same as input  ParamDataTypeStr=Inherit: Same as input
  Saturation : Saturate  UpperLimit=LimitU_Ireg_stat  LowerLimit=LimitL_Ireg_stat
  Sum : Sum  Inputs=|-+
  Sum1 : Sum  Inputs=|-+
  VdVq_conv : Outport  VectorParamsAs1DForOutWhenUnconnected=off
  wires:
  Add3/1 -> Correction to VdVq due to delays + Transfo Connection/2(Vq)
  Add1/1 -> Correction to VdVq due to delays + Transfo Connection/1(Vd)  "Feedforward"
  PI_d/1(Out) -> [PId], Add1/2
  PI_q/1(Out) -> [PIq], Add3/2
  [Vd] -> Add1/1
  Product1/1 -> Add1/4
  Gain/1 -> Add1/3
  Gain1/1 -> Add3/3
  Product2/1 -> Add3/4
  [Vq] -> Add3/1
  Demux2/1 -> [Id]
  IdIq/1 -> Demux2/1
  [Id_ref] -> Product2/1
  [Iq_ref] -> Gain1/1
  [Iq_ref] -> Product1/1
  [Id_ref] -> Gain/1
  Saturation/1 -> VdVq_conv/1
  [Id] -> Sum/1
  [Iq] -> Sum1/1
  Demux2/2 -> [Iq]
  Correction to VdVq due to delays + Transfo Connection/2(Vq*) -> Mux/2
  Correction to VdVq due to delays + Transfo Connection/1(Vd*) -> Mux/1
  [PIq] -> Mux1/2
  [PId] -> Mux1/1
  [w] -> Product1/3
  Constant2/1 -> Product1/2
  [w] -> Product2/3
  Constant1/1 -> Product2/2
  Mux1/1 -> PI_Ireg/1
  [Iq_ref] -> Sum1/2
  Sum1/1 -> PI_q/1(Error)
  [Id_ref] -> Sum/2
  Sum/1 -> PI_d/1(Error)
  Mux/1 -> Saturation/1
  VdVq/1 -> Demux3/1
  Demux3/2 -> [Vq]
  Demux3/1 -> [Vd]
  IdIq_ref/1 -> Demux1/1
  Demux1/2 -> [Iq_ref]
  Demux1/1 -> [Id_ref]
  Rtot_pu3/1 -> [w]
  Freq/1 -> Rtot_pu3/1

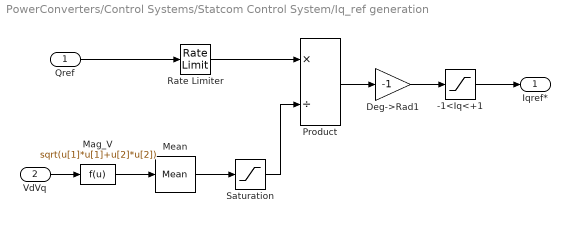
== system PowerConverters/Control Systems/Statcom Control System/Iq_ref generation ==
  Qref : Inport  PortDimensions=1
  VdVq : Inport  Port=2  PortDimensions=2
  -1<Iq<+1 : Saturate  UpperLimit=1  LowerLimit=-1
  Deg->Rad1 : Gain  Gain=-1  SaturateOnIntegerOverflow=on  OutDataTypeStr=Inherit: Same as input  ParamDataTypeStr=Inherit: Same as input
  "Mag_V " : Fcn  Expr=sqrt(u[1]*u[1]+u[2]*u[2])
  Mean : spsMeanLib/Mean  Freq=Fnom  Vinit=1  Ts=Ts_Control
  Product : Product  Inputs=*/  InputSameDT=on  SaturateOnIntegerOverflow=on  OutDataTypeStr=Inherit: Same as first input
  Rate Limiter : RateLimiter  RisingSlewLimit=RateLimit_Qstat  FallingSlewLimit=-RateLimit_Qstat  SampleTimeMode=inherited
      settings: AttributesFormatString=Up = %<RisingSlewLimit>\nDown = %<FallingSlewLimit>
  Saturation : Saturate  UpperLimit=inf  LowerLimit=eps
  Iqref* : Outport  VectorParamsAs1DForOutWhenUnconnected=off
  wires:
  Mean/1 -> Saturation/1
  VdVq/1 -> "Mag_V "/1
  "Mag_V "/1 -> Mean/1
  Saturation/1 -> Product/2
  Product/1 -> Deg->Rad1/1
  Deg->Rad1/1 -> -1<Iq<+1/1
  -1<Iq<+1/1 -> Iqref*/1
  Qref/1 -> Rate Limiter/1
  Rate Limiter/1 -> Product/1

== system PowerConverters/Control Systems/Statcom Control System/Measurements ==
  Vabc : Inport  PortDimensions=3
  PLL (3ph) : spsPLL3phLib/PLL (3ph)  Fmin=45  Par_Init=[0, Fnom]  ParK=[180, 3200, 0]/2  TcD=1e-4  MaxRateChangeFreq=12  FilterCutOffFreq=25  Ts=Ts_Control  AGC=on
  Selector2 : Selector  InputPortWidth=3  IndexOptions=Index vector (dialog)  Indices=[1 2]  OutputSizes=1
  V->pu1 : Gain  Gain=1/(Vnom_prim_stat*sqrt(2)/sqrt(3))  SaturateOnIntegerOverflow=on  OutDataTypeStr=Inherit: Same as input  ParamDataTypeStr=Inherit: Same as input
  abc to dq1 : spsabctodq0Lib/abc to dq0  Alignment=90 degrees behind phase A axis
  wt : Outport  VectorParamsAs1DForOutWhenUnconnected=off
  VdVq : Outport  Port=2  VectorParamsAs1DForOutWhenUnconnected=off
  Freq : Outport  Port=3  VectorParamsAs1DForOutWhenUnconnected=off
  wires:
  Selector2/1 -> VdVq/1
  abc to dq1/1 -> Selector2/1
  PLL (3ph)/1 -> Freq/1
  V->pu1/1 -> PLL (3ph)/1, abc to dq1/1
  Vabc/1 -> V->pu1/1
  PLL (3ph)/2 -> wt/1, abc to dq1/2

== system PowerConverters/Control Systems/Statcom Control System/Scaling ==
  Vdc : Inport
  VdVq : Inport  Port=2
  0.5 to 1.5 x Vnom_dc : Saturate  UpperLimit=1.5*Vnom_dc_stat  LowerLimit=0.5*Vnom_dc_stat
  Constant2 : Constant  Value=Vnom_sec_stat/sqrt(3)*sqrt(2)
  Gain1 : Gain
  Product : Product  Inputs=*/
  Product1 : Product  Inputs=**
  VdVq* : Outport  VectorParamsAs1DForOutWhenUnconnected=off
  wires:
  Product1/1 -> VdVq*/1
  VdVq/1 -> Product1/1
  Vdc/1 -> 0.5 to 1.5 x Vnom_dc/1
  Product/1 -> Product1/2
  0.5 to 1.5 x Vnom_dc/1 -> Gain1/1
  Gain1/1 -> Product/2
  Constant2/1 -> Product/1

== system PowerConverters/Control Systems/Statcom Control System/VDC Regulator (VDCreg) ==
  Vdc : Inport  PortDimensions=1
  Vdc_ref : Inport  Port=2  PortDimensions=1
  Gain : Gain  Gain=1/(Vnom_dc_stat)
  PI_d : Subsystem  DialogController=POWERSYS.PowerSysDialog  mask(Discrete PI Controller){Kp=Kp_VDCreg_stat, Ki=Ki_VDCreg_stat, Par_Limits=[ LimitU_VDCreg_stat,  LimitL_VDCreg_stat ], Init=0, Ts=Ts_Control}
      mask prompts: Kp "Proportional gain (Kp):"; Ki "Integral gain (Ki):"; Par_Limits "Output limits: [ Upper   Lower ]"; Init "Output initial value:"; Ts "Sample time:"
      mask help: This block implements a discrete PI controller.
      mask init:
      | UpperLimit=Par_Limits(1);
      | LowerLimit=Par_Limits(2);
      mask Display: disp('PI');
  Sum : Sum  Inputs=|-+
  Idref : Outport  VectorParamsAs1DForOutWhenUnconnected=off
  wires:
  PI_d/1(Out) -> Idref/1
  Gain/1 -> PI_d/1(Error)
  Vdc/1 -> Sum/2
  Vdc_ref/1 -> Sum/1
  Sum/1 -> Gain/1

== system PowerConverters/Control Systems/PWM Gen 3L/PWMgen - Averaging/Subsystem ==
  Uref : Inport
  PWM Gen 3L : spsPWMGenerator3LevelLib/PWM Generator (3-Level)  ModulatorType=Three-phase bridge (12 pulses)  ModulatorMode=Unsynchronized  nF=27  Fc=Fc_3L  ModulatingSignals=off  m=0.8  Freq=60  Phase=0  Ts=Ts_PWM
  P : Outport
  wires:
  Uref/1 -> PWM Gen 3L/1
  PWM Gen 3L/1 -> P/1

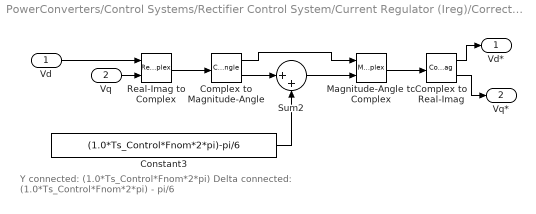
== system PowerConverters/Control Systems/Rectifier Control System/Current Regulator (Ireg)/Correction to VdVq due to delays + Transfo Connection ==
  note: Y connected: (1.0*Ts_Control*Fnom*2*pi)
      | Delta connected: (1.0*Ts_Control*Fnom*2*pi) - pi/6
  Vd : Inport
  Vq : Inport  Port=2
  Complex to Magnitude-Angle : ComplexToMagnitudeAngle
  Complex to Real-Imag : ComplexToRealImag
  Constant3 : Constant  Value=(1.0*Ts_Control*Fnom*2*pi)-pi/6  SampleTime=Ts_Control
  Magnitude-Angle to Complex : MagnitudeAngleToComplex
  Real-Imag to Complex : RealImagToComplex
  Sum2 : Sum  Inputs=|++
  Vd* : Outport  VectorParamsAs1DForOutWhenUnconnected=off
  Vq* : Outport  Port=2  VectorParamsAs1DForOutWhenUnconnected=off
  wires:
  Constant3/1 -> Sum2/2
  Complex to Magnitude-Angle/2 -> Sum2/1
  Magnitude-Angle to Complex/1 -> Complex to Real-Imag/1
  Sum2/1 -> Magnitude-Angle to Complex/2
  Real-Imag to Complex/1 -> Complex to Magnitude-Angle/1
  Complex to Magnitude-Angle/1 -> Magnitude-Angle to Complex/1
  Complex to Real-Imag/1 -> Vd*/1
  Vq/1 -> Real-Imag to Complex/2
  Vd/1 -> Real-Imag to Complex/1
  Complex to Real-Imag/2 -> Vq*/1

== system PowerConverters/Control Systems/Rectifier Control System/Current Regulator (Ireg)/PI_d ==
  Error : Inport  SampleTime=Ts
  Discrete-Time Integrator : DiscreteIntegrator  InitialCondition=Init  SampleTime=Ts  LimitOutput=on  UpperSaturationLimit=UpperLimit  LowerSaturationLimit=LowerLimit  ICPrevOutput=DiscIntNeverNeededParam  ICPrevScaledInput=DiscIntNeverNeededParam
  Kp4 : Gain  Gain=Kp  SaturateOnIntegerOverflow=on  SampleTime=Ts  OutDataTypeStr=Inherit: Same as input  ParamDataTypeStr=Inherit: Same as input
  Kp5 : Gain  Gain=Ki  SaturateOnIntegerOverflow=on  SampleTime=Ts  OutDataTypeStr=Inherit: Same as input  ParamDataTypeStr=Inherit: Same as input
  Saturation2 : Saturate  UpperLimit=UpperLimit  LowerLimit=LowerLimit  SampleTime=Ts
  Sum6 : Sum  InputSameDT=on  SaturateOnIntegerOverflow=on  SampleTime=Ts  OutDataTypeStr=Inherit: Same as first input
  Zero-Order Hold : ZeroOrderHold  SampleTime=Ts
  Out : Outport  SampleTime=Ts  InitialOutput=0  VectorParamsAs1DForOutWhenUnconnected=off
  wires:
  Saturation2/1 -> Out/1
  Error/1 -> Kp4/1, Kp5/1
  Sum6/1 -> Saturation2/1
  Kp5/1 -> Discrete-Time Integrator/1
  Kp4/1 -> Zero-Order Hold/1
  Discrete-Time Integrator/1 -> Sum6/2
  Zero-Order Hold/1 -> Sum6/1

== system PowerConverters/Control Systems/Rectifier Control System/Current Regulator (Ireg)/PI_q ==
  Error : Inport  SampleTime=Ts
  Discrete-Time Integrator : DiscreteIntegrator  InitialCondition=Init  SampleTime=Ts  LimitOutput=on  UpperSaturationLimit=UpperLimit  LowerSaturationLimit=LowerLimit  ICPrevOutput=DiscIntNeverNeededParam  ICPrevScaledInput=DiscIntNeverNeededParam
  Kp4 : Gain  Gain=Kp  SaturateOnIntegerOverflow=on  SampleTime=Ts  OutDataTypeStr=Inherit: Same as input  ParamDataTypeStr=Inherit: Same as input
  Kp5 : Gain  Gain=Ki  SaturateOnIntegerOverflow=on  SampleTime=Ts  OutDataTypeStr=Inherit: Same as input  ParamDataTypeStr=Inherit: Same as input
  Saturation2 : Saturate  UpperLimit=UpperLimit  LowerLimit=LowerLimit  SampleTime=Ts
  Sum6 : Sum  InputSameDT=on  SaturateOnIntegerOverflow=on  SampleTime=Ts  OutDataTypeStr=Inherit: Same as first input
  Zero-Order Hold : ZeroOrderHold  SampleTime=Ts
  Out : Outport  SampleTime=Ts  InitialOutput=0  VectorParamsAs1DForOutWhenUnconnected=off
  wires:
  Zero-Order Hold/1 -> Sum6/1
  Discrete-Time Integrator/1 -> Sum6/2
  Kp4/1 -> Zero-Order Hold/1
  Kp5/1 -> Discrete-Time Integrator/1
  Sum6/1 -> Saturation2/1
  Error/1 -> Kp5/1, Kp4/1
  Saturation2/1 -> Out/1

== system PowerConverters/Control Systems/Rectifier Control System/VDC Regulator (VDCreg)/PI_d ==
  Error : Inport  SampleTime=Ts
  Discrete-Time Integrator : DiscreteIntegrator  InitialCondition=Init  SampleTime=Ts  LimitOutput=on  UpperSaturationLimit=UpperLimit  LowerSaturationLimit=LowerLimit  ICPrevOutput=DiscIntNeverNeededParam  ICPrevScaledInput=DiscIntNeverNeededParam
  Kp4 : Gain  Gain=Kp  SaturateOnIntegerOverflow=on  SampleTime=Ts  OutDataTypeStr=Inherit: Same as input  ParamDataTypeStr=Inherit: Same as input
  Kp5 : Gain  Gain=Ki  SaturateOnIntegerOverflow=on  SampleTime=Ts  OutDataTypeStr=Inherit: Same as input  ParamDataTypeStr=Inherit: Same as input
  Saturation2 : Saturate  UpperLimit=UpperLimit  LowerLimit=LowerLimit  SampleTime=Ts
  Sum6 : Sum  InputSameDT=on  SaturateOnIntegerOverflow=on  SampleTime=Ts  OutDataTypeStr=Inherit: Same as first input
  Zero-Order Hold : ZeroOrderHold  SampleTime=Ts
  Out : Outport  SampleTime=Ts  InitialOutput=0  VectorParamsAs1DForOutWhenUnconnected=off
  wires:
  Saturation2/1 -> Out/1
  Error/1 -> Kp4/1, Kp5/1
  Sum6/1 -> Saturation2/1
  Kp5/1 -> Discrete-Time Integrator/1
  Kp4/1 -> Zero-Order Hold/1
  Discrete-Time Integrator/1 -> Sum6/2
  Zero-Order Hold/1 -> Sum6/1

== system PowerConverters/Control Systems/Statcom Control System/Current Regulator (Ireg)/Correction to VdVq due to delays + Transfo Connection ==
  note: Y connected: (1.0*Ts_Control*Fnom*2*pi)
      | Delta connected: (1.0*Ts_Control*Fnom*2*pi) - pi/6
  Vd : Inport
  Vq : Inport  Port=2
  Complex to Magnitude-Angle : ComplexToMagnitudeAngle
  Complex to Real-Imag : ComplexToRealImag
  Constant3 : Constant  Value=(1.0*Ts_Control*Fnom*2*pi)  SampleTime=Ts_Control
  Magnitude-Angle to Complex : MagnitudeAngleToComplex
  Real-Imag to Complex : RealImagToComplex
  Sum2 : Sum  Inputs=|++
  Vd* : Outport  VectorParamsAs1DForOutWhenUnconnected=off
  Vq* : Outport  Port=2  VectorParamsAs1DForOutWhenUnconnected=off
  wires:
  Constant3/1 -> Sum2/2
  Complex to Magnitude-Angle/2 -> Sum2/1
  Magnitude-Angle to Complex/1 -> Complex to Real-Imag/1
  Sum2/1 -> Magnitude-Angle to Complex/2
  Real-Imag to Complex/1 -> Complex to Magnitude-Angle/1
  Complex to Magnitude-Angle/1 -> Magnitude-Angle to Complex/1
  Complex to Real-Imag/1 -> Vd*/1
  Vq/1 -> Real-Imag to Complex/2
  Vd/1 -> Real-Imag to Complex/1
  Complex to Real-Imag/2 -> Vq*/1

== system PowerConverters/Control Systems/Statcom Control System/Current Regulator (Ireg)/PI_d ==
  Error : Inport  SampleTime=Ts
  Discrete-Time Integrator : DiscreteIntegrator  InitialCondition=Init  SampleTime=Ts  LimitOutput=on  UpperSaturationLimit=UpperLimit  LowerSaturationLimit=LowerLimit  ICPrevOutput=DiscIntNeverNeededParam  ICPrevScaledInput=DiscIntNeverNeededParam
  Kp4 : Gain  Gain=Kp  SaturateOnIntegerOverflow=on  SampleTime=Ts  OutDataTypeStr=Inherit: Same as input  ParamDataTypeStr=Inherit: Same as input
  Kp5 : Gain  Gain=Ki  SaturateOnIntegerOverflow=on  SampleTime=Ts  OutDataTypeStr=Inherit: Same as input  ParamDataTypeStr=Inherit: Same as input
  Saturation2 : Saturate  UpperLimit=UpperLimit  LowerLimit=LowerLimit  SampleTime=Ts
  Sum6 : Sum  InputSameDT=on  SaturateOnIntegerOverflow=on  SampleTime=Ts  OutDataTypeStr=Inherit: Same as first input
  Zero-Order Hold : ZeroOrderHold  SampleTime=Ts
  Out : Outport  SampleTime=Ts  InitialOutput=0  VectorParamsAs1DForOutWhenUnconnected=off
  wires:
  Saturation2/1 -> Out/1
  Error/1 -> Kp4/1, Kp5/1
  Sum6/1 -> Saturation2/1
  Kp5/1 -> Discrete-Time Integrator/1
  Kp4/1 -> Zero-Order Hold/1
  Discrete-Time Integrator/1 -> Sum6/2
  Zero-Order Hold/1 -> Sum6/1

== system PowerConverters/Control Systems/Statcom Control System/Current Regulator (Ireg)/PI_q ==
  Error : Inport  SampleTime=Ts
  Discrete-Time Integrator : DiscreteIntegrator  InitialCondition=Init  SampleTime=Ts  LimitOutput=on  UpperSaturationLimit=UpperLimit  LowerSaturationLimit=LowerLimit  ICPrevOutput=DiscIntNeverNeededParam  ICPrevScaledInput=DiscIntNeverNeededParam
  Kp4 : Gain  Gain=Kp  SaturateOnIntegerOverflow=on  SampleTime=Ts  OutDataTypeStr=Inherit: Same as input  ParamDataTypeStr=Inherit: Same as input
  Kp5 : Gain  Gain=Ki  SaturateOnIntegerOverflow=on  SampleTime=Ts  OutDataTypeStr=Inherit: Same as input  ParamDataTypeStr=Inherit: Same as input
  Saturation2 : Saturate  UpperLimit=UpperLimit  LowerLimit=LowerLimit  SampleTime=Ts
  Sum6 : Sum  InputSameDT=on  SaturateOnIntegerOverflow=on  SampleTime=Ts  OutDataTypeStr=Inherit: Same as first input
  Zero-Order Hold : ZeroOrderHold  SampleTime=Ts
  Out : Outport  SampleTime=Ts  InitialOutput=0  VectorParamsAs1DForOutWhenUnconnected=off
  wires:
  Zero-Order Hold/1 -> Sum6/1
  Discrete-Time Integrator/1 -> Sum6/2
  Kp4/1 -> Zero-Order Hold/1
  Kp5/1 -> Discrete-Time Integrator/1
  Sum6/1 -> Saturation2/1
  Error/1 -> Kp5/1, Kp4/1
  Saturation2/1 -> Out/1

== system PowerConverters/Control Systems/Statcom Control System/VDC Regulator (VDCreg)/PI_d ==
  Error : Inport  SampleTime=Ts
  Discrete-Time Integrator : DiscreteIntegrator  InitialCondition=Init  SampleTime=Ts  LimitOutput=on  UpperSaturationLimit=UpperLimit  LowerSaturationLimit=LowerLimit  ICPrevOutput=DiscIntNeverNeededParam  ICPrevScaledInput=DiscIntNeverNeededParam
  Kp4 : Gain  Gain=Kp  SaturateOnIntegerOverflow=on  SampleTime=Ts  OutDataTypeStr=Inherit: Same as input  ParamDataTypeStr=Inherit: Same as input
  Kp5 : Gain  Gain=Ki  SaturateOnIntegerOverflow=on  SampleTime=Ts  OutDataTypeStr=Inherit: Same as input  ParamDataTypeStr=Inherit: Same as input
  Saturation2 : Saturate  UpperLimit=UpperLimit  LowerLimit=LowerLimit  SampleTime=Ts
  Sum6 : Sum  InputSameDT=on  SaturateOnIntegerOverflow=on  SampleTime=Ts  OutDataTypeStr=Inherit: Same as first input
  Zero-Order Hold : ZeroOrderHold  SampleTime=Ts
  Out : Outport  SampleTime=Ts  InitialOutput=0  VectorParamsAs1DForOutWhenUnconnected=off
  wires:
  Saturation2/1 -> Out/1
  Error/1 -> Kp4/1, Kp5/1
  Sum6/1 -> Saturation2/1
  Kp5/1 -> Discrete-Time Integrator/1
  Kp4/1 -> Zero-Order Hold/1
  Discrete-Time Integrator/1 -> Sum6/2
  Zero-Order Hold/1 -> Sum6/1
